simulink model "Versuch 1"  (R2022b)
settings: Solver=VariableStepAuto  StartTime=0.0  StopTime=10.0  RelTol=1e-3
settings Model: Creator=janne  LastModifiedBy=janne

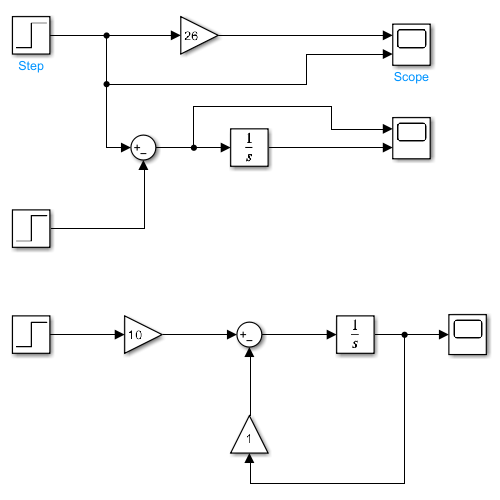
[thumbnail: Simulink's stored preview of the top-level diagram]
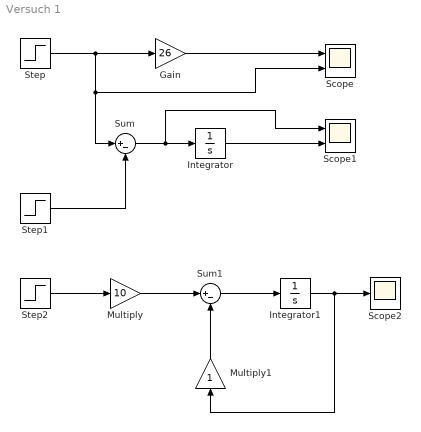
== system Versuch 1 ==
  Gain : Gain  Gain=26
  Integrator : Integrator
  Integrator1 : Integrator
  Multiply : Gain  Gain=10
  Multiply1 : Gain
  Scope : Scope  NumInputPorts=2
  Scope1 : Scope  NumInputPorts=2
  Scope2 : Scope
  Step : Step  SampleTime=0
  Step1 : Step  Time=4  SampleTime=0
  Step2 : Step  SampleTime=0
  Sum : Sum  Inputs=|+-
  Sum1 : Sum  Inputs=|+-
  wires:
  Gain/1 -> Scope/1
  Step/1 -> Scope/2, Sum/1, Gain/1
  Step1/1 -> Sum/2
  Sum/1 -> Scope1/1, Integrator/1
  Integrator/1 -> Scope1/2
  Multiply/1 -> Sum1/1
  Multiply1/1 -> Sum1/2
  Sum1/1 -> Integrator1/1
  Integrator1/1 -> Scope2/1, Multiply1/1
  Step2/1 -> Multiply/1
